simulink model "playback_data"  (R2015a)
settings: Solver=FixedStepDiscrete  SolverMode=SingleTasking  StartTime=76  StopTime=110  FixedStep=sample_time  RelTol=1e-3
undefined symbols (not defined in the file): A1_notch_f1, A2_notch_f1, A_kalman_swing_load, A_kalman_transverse, A_kalman_vertical, A_lpf_accelerometer, A_lpf_dtau, A_lpf_fourbar_angles, A_lpf_imu, A_lpf_lateral_angle, B1_lpf_accelerometer, B1_lpf_dtau, B1_lpf_fourbar_angles, B1_lpf_imu, B1_lpf_lateral_angle, B1_notch_f1, B2_lpf_accelerometer, B2_lpf_dtau, B2_lpf_fourbar_angles, B2_lpf_imu, B2_lpf_lateral_angle, B2_notch_f1, B_dx_versus_x0, B_kalman_swing_load, B_kalman_transverse, B_kalman_vertical, backwards_K_sag_of_t, backwards_P_sag_of_t, C_kalman_swing_load, C_kalman_transverse, C_kalman_vertical, com_leg_motor, com_torso, contact_threshold, control_start_time, d_ankle_to_foot, d_vertical_com, desired_com_forward_velocity, desired_com_lateral_velocity, desired_initial_leg_roll_left, desired_initial_leg_roll_right, desired_stance_beta2, desired_standing_torso_pitch, desired_standing_torso_roll, desired_standing_z, desired_torso_pitch, desired_torso_roll, Discrete, enable_bouncing, fcut_contact, fdesignblkfcn, forward_dx_of_dxstar, forward_x_of_dxstar, g, gcbh, HIP_MTR_MAX_CONT_TORQUE, HIP_MTR_MAX_TORQUE, i_leg_motor, i_robot, i_torso ... (+78)
libraries: simulink x65, dsparch4 x18, ctrlSharedLib x14, dspfdesign x4
(part 10 of 13)

== matlab function playback_data/Control/Actuator Control with Torque SEA commands/Detect Collision ==
  data: time input; spring_torque input; load_torque_derivative input; in_collision output; swing_collision_wait_time parameter
function in_collision = detect_collision(time, spring_torque, load_torque_derivative, swing_collision_wait_time)
    
    persistent collision_state time_of_collision;
    if isempty(collision_state)
        collision_state = logical(zeros(4,1));
        time_of_collision = zeros(4,1);
    end

    collision_detected = (abs(load_torque_derivative) > 2000 | abs(spring_torque) >= 50) & (time - time_of_collision > (1.5*swing_collision_wait_time));
    time_of_collision(collision_detected) = time;
    collision_state = collision_state | collision_detected;
    time_since_collision = time - time_of_collision;
    out_of_collision = (time_since_collision > swing_collision_wait_time) & (abs(spring_torque) < 50);
    collision_state(out_of_collision) = 0;
    %in_collision = collision_state;
    in_collision = [collision_state(1) | collision_state(2);
                    collision_state(1) | collision_state(2);
                    collision_state(3) | collision_state(4);
                    collision_state(3) | collision_state(4)];
    
end

== matlab function playback_data/Control/Actuator Control with Torque SEA commands/Load Torque Kalman Filter/MATLAB Function ==
  data: spring_torques input; R1 output; sample_time parameter; R2 output; R3 output; R4 output
function [R1, R2, R3, R4] = MeasurementCovariance(spring_torques, sample_time)
         
    high_torque_threshold = 80;
    low_torque_threshold = 50;
    high_deviation = 10;
    low_deviation = 0.1;
    
    deviation = (abs(spring_torques)-low_torque_threshold)*(low_deviation-high_deviation)/(high_torque_threshold-low_torque_threshold) + high_deviation;
    deviation(abs(spring_torques) <= low_torque_threshold) = high_deviation;
    deviation(abs(spring_torques) >= high_torque_threshold) = low_deviation;

    R1 = diag([(1e-6)^2, deviation(1)^2])/sample_time;
    R2 = diag([(1e-6)^2, deviation(2)^2])/sample_time;
    R3 = diag([(1e-6)^2, deviation(3)^2])/sample_time;
    R4 = diag([(1e-6)^2, deviation(4)^2])/sample_time;
end

== matlab function playback_data/Control/Actuator Control with Torque SEA commands/SEA Controller (Velocity)/Nonlinear Spring Force ==
  data: deflections input; tau_sea output
function tau_sea   = SeaSpringForce( deflections )
    tau_sea = SeaSpringForce( deflections );
end

== matlab function playback_data/Control/Behavior Control/Compute COM Translational Acceleration (IMU uses non-rotating measurement frame) ==
  data: com_acceleration_world output; torso_angular_accelerations input; imu_translational_accelerations_body input; torso_roll input; torso_pitch input; torso_yaw input; com_position_world input; com_velocity_world input; hip_roll_accelerations input; right_hip_roll input; left_hip_roll input; pelvis_to_imu parameter; com_torso parameter; com_leg_motor parameter; m_leg_motor parameter; m_leg parameter; m_torso parameter; torso_com_acceleration_world output; pelvis_acceleration_world output; right_hip_acceleration_world output; left_hip_acceleration_world output; com_acceleration_yawed output; g parameter
function [com_acceleration_world, torso_com_acceleration_world, pelvis_acceleration_world, right_hip_acceleration_world, left_hip_acceleration_world, com_acceleration_yawed] ...
          = compute_com_acceleration(torso_angular_accelerations, imu_translational_accelerations_body, torso_roll, torso_pitch, torso_yaw, ...
          com_position_world, com_velocity_world, ...
          hip_roll_accelerations, right_hip_roll, left_hip_roll, pelvis_to_imu, com_torso, com_leg_motor, m_leg_motor, m_leg, m_torso, g)

    % Body frame to Yawed frame rotations  
    R_body_to_yawed = R_pitch(torso_pitch(1))*R_roll(torso_roll(1));
    dR_body_to_yawed = dR_pitch(torso_pitch(1),torso_pitch(2))*R_roll(torso_roll(1)) + R_pitch(torso_pitch(1))*dR_roll(torso_roll(1),torso_roll(2));
    ddR_body_to_yawed = ddR_pitch(torso_pitch(1),torso_pitch(2),torso_angular_accelerations(2))*R_roll(torso_roll(1)) ...
                        + R_pitch(torso_pitch(1))*ddR_roll(torso_roll(1),torso_roll(2),torso_angular_accelerations(1)) ... 
                        + 2*dR_pitch(torso_pitch(1),torso_pitch(2))*dR_roll(torso_roll(1),torso_roll(2));
    % Yawed frame to World frame rotations  
    R_yawed_to_world = R_yaw(torso_yaw(1));
    dR_yawed_to_world = dR_yaw(torso_yaw(1),torso_yaw(2));
    ddR_yawed_to_world = ddR_yaw(torso_yaw(1),torso_yaw(2),torso_angular_accelerations(3));
    % Compute translational acceleration of torso COM
    R_position_body_to_world = R_yawed_to_world*R_body_to_yawed;
    R_velocity_body_to_world = dR_yawed_to_world*R_body_to_yawed + R_yawed_to_world*dR_body_to_yawed;
    R_acceleration_body_to_world = ddR_yawed_to_world*R_body_to_yawed + 2*dR_yawed_to_world*dR_body_to_yawed + R_yawed_to_world*ddR_body_to_yawed;
    imu_to_torso_com_acceleration_world = R_acceleration_body_to_world*(com_torso - pelvis_to_imu)';
    imu_acceleration_world = R_yawed_to_world*R_body_to_yawed*imu_translational_accelerations_body;
    torso_com_acceleration_world = imu_acceleration_world + imu_to_torso_com_acceleration_world;
    % Compute accelerations of hip COMs
    R_right_hip_to_body =     R_roll(-pi/2+right_hip_roll(1));
    dR_right_hip_to_body =   dR_roll(-pi/2+right_hip_roll(1), right_hip_roll(2));
    ddR_right_hip_to_body = ddR_roll(-pi/2+right_hip_roll(1), right_hip_roll(2), hip_roll_accelerations(1));
    R_left_hip_to_body =     R_roll(pi/2-left_hip_roll(1));
    dR_left_hip_to_body =   dR_roll(pi/2-left_hip_roll(1), -left_hip_roll(2));
    ddR_left_hip_to_body = ddR_roll(pi/2-left_hip_roll(1), -left_hip_roll(2), -hip_roll_accelerations(2));
    imu_to_pelvis_com_acceleration_world = R_acceleration_body_to_world*(-pelvis_to_imu)';  
    pelvis_acceleration_world = imu_acceleration_world + imu_to_pelvis_com_acceleration_world;
    left_hip_acceleration_world = pelvis_acceleration_world + (R_acceleration_body_to_world*R_left_hip_to_body + 2*R_velocity_body_to_world*dR_left_hip_to_body + R_position_body_to_world*ddR_left_hip_to_body)*com_leg_motor';
    right_hip_acceleration_world = pelvis_acceleration_world + (R_acceleration_body_to_world*R_right_hip_to_body + 2*R_velocity_body_to_world*dR_right_hip_to_body + R_position_body_to_world*ddR_right_hip_to_body)*(com_leg_motor.*[1,-1,1])';
    % Compute total system COM acceleration
    m_hip = m_leg+m_leg_motor;
    m_total = 2*m_hip + m_torso;
    com_acceleration_world = (m_torso*torso_com_acceleration_world + m_hip*(left_hip_acceleration_world + right_hip_acceleration_world))/m_total;
    com_acceleration_yawed = ddR_yawed_to_world'*com_position_world + 2*dR_yawed_to_world'*com_velocity_world + R_yawed_to_world'*com_acceleration_world;
    com_acceleration_yawed(3) = com_acceleration_yawed(3) - g;
end

function R_yp = R_pitch(theta) % map from pitched to yawed
  R_yp = [cos(theta), 0, sin(theta); ...
          0, 1, 0; ...
          -sin(theta), 0, cos(theta)];
end
function dR_yp = dR_pitch(theta,dtheta)
  dR_yp = dtheta*[-sin(theta), 0, cos(theta); ...
                  0, 0, 0; ... 
                  -cos(theta), 0, -sin(theta)];
end
function ddR_yp = ddR_pitch(theta,dtheta,ddtheta)
  ddR_yp = ddtheta*[-sin(theta), 0, cos(theta); ...
                    0, 0, 0; ... 
                    -cos(theta), 0, -sin(theta)] ...
           + dtheta^2*[-cos(theta), 0, -sin(theta); ...
                     0, 0, 0; ...
                     sin(theta), 0, -cos(theta)];
end
function R_pr = R_roll(phi) % map from rolled to pitched
  R_pr = [1, 0, 0; ...
          0, cos(phi), -sin(phi); ...
          0, sin(phi), cos(phi)]; 
end
function dR_pr = dR_roll(phi,dphi)
  dR_pr = dphi*[0, 0, 0; ...
                0, -sin(phi), -cos(phi); ...
                0, cos(phi), -sin(phi)];
end
function ddR_pr = ddR_roll(phi, dphi, ddphi)
  ddR_pr = ddphi*[0, 0, 0; ...
                  0, -sin(phi), -cos(phi); ...
                  0, cos(phi), -sin(phi)] ...
           + dphi^2*[0, 0, 0; ...
                   0, -cos(phi), sin(phi);...
                   0, -sin(phi), -cos(phi)];
end
function R_gy = R_yaw(psi) % map yawed frame to global
  R_gy = [cos(psi), -sin(psi), 0; sin(psi), cos(psi), 0; 0 0 1]; 
end
function dR_gy = dR_yaw(psi,dpsi)
  dR_gy = dpsi*[-sin(psi), -cos(psi), 0; cos(psi), -sin(psi), 0; 0 0 0];
end
function ddR_gy = ddR_yaw(psi,dpsi,ddpsi)
  ddR_gy = ddpsi*[-sin(psi), -cos(psi), 0; cos(psi), -sin(psi), 0; 0 0 0] ...
           + dpsi^2*[-cos(psi), sin(psi), 0; -sin(psi), -cos(psi), 0; 0 0 0];
end

== matlab function playback_data/Control/Behavior Control/Compute World Frame COM Coordinates from Yawed Frame ==
  data: com_position_world output; X_dX input; Y_dY input; Z_dZ input; torso_yaw input; com_velocity_world output
function [com_position_world, com_velocity_world] ...
          = compute_com_state_in_world_frame(X_dX, Y_dY, Z_dZ, torso_yaw)

    R_yawed_to_world = R_yaw(torso_yaw(1));
    dR_yawed_to_world = dR_yaw(torso_yaw(1),torso_yaw(2));
    
    com_position_yawed = [X_dX(1); Y_dY(1); Z_dZ(1)];
    com_velocity_yawed = [X_dX(2); Y_dY(2); Z_dZ(2)];
    
    com_position_world = R_yawed_to_world*com_position_yawed;
    com_velocity_world = dR_yawed_to_world*com_position_yawed + R_yawed_to_world*com_velocity_yawed;

end

function R_gy = R_yaw(psi) % map yawed frame to global
  R_gy = [cos(psi), -sin(psi), 0; sin(psi), cos(psi), 0; 0 0 1]; 
end
function dR_gy = dR_yaw(psi,dpsi)
  dR_gy = dpsi*[-sin(psi), -cos(psi), 0; cos(psi), -sin(psi), 0; 0 0 0];
end

== stateflow chart playback_data/Control/Behavior Control/Contact State Machine/State Machine ==
  state TouchDown
  state LockedContact
  state Unloading
  state Takeoff
  state Flight
  (junction 91) -> TouchDown
  TouchDown -> (junction 130) [order 2] : [vertical_grf < contact_threshold]
  (junction 93) -> (junction 91)
  (junction 130) -> (junction 128)
  TouchDown -> LockedContact [order 1] : [vertical_grf > loaded_threshold]
  (junction 115) -> LockedContact
  (junction 118) -> (junction 115)
  LockedContact -> Unloading : [z_velocity >= 0 && previous_z_velocity < 0]
  Unloading -> LockedContact [order 2] : [vertical_grf > loaded_threshold && z_velocity < 0]
  (junction 122) -> (junction 118)
  Unloading -> Takeoff [order 1] : [vertical_grf < contact_threshold]
  Takeoff -> Flight : after(t_flight,sec)
  (default) -> Flight
  Flight -> (junction 93) : [vertical_grf > contact_threshold]
  (junction 128) -> Flight
  data: z_velocity input; previous_z_velocity input; vertical_grf input; t_flight parameter; g parameter; contact_threshold parameter; loaded_threshold parameter; TouchDown output boolean; LockedContact output boolean; Unloading output boolean; Takeoff output boolean; Flight output boolean; vertical_acceleration input

== matlab function playback_data/Control/Behavior Control/Force Estimation/3D Forward Dynamics yawed ==
  data: right_or_left input; torso_roll input size=2; torso_pitch input double size=2; torso_yaw input double size=2; primary_sagittal_leg_angle input double size=2; primary_leg_length input double size=2; primary_leg_roll input double size=2; secondary_leg_roll input double size=2; primary_leg_torque input; primary_leg_force input; primary_lateral_torque input; secondary_lateral_torque input; R_GRF output double size=3; L_GRF output size=3; ddroll output double; g parameter; m_leg_motor parameter; m_torso parameter; i_torso parameter; i_leg_motor parameter; lateral_offset parameter; com_torso parameter; torso_centerline_roll_offset_angle parameter
%% Forward 3D ATRIAS dynamics
function [R_GRF, L_GRF, ddroll]  =  ForwardDynamics3D(right_or_left, ...
                                                      torso_roll, torso_pitch, torso_yaw, ...
                                                      primary_sagittal_leg_angle, primary_leg_length,...
                                                      primary_leg_roll, secondary_leg_roll, ...
                                                      primary_leg_torque, primary_leg_force, ...
                                                      primary_lateral_torque, secondary_lateral_torque, ...
                                                      g, m_leg_motor, m_torso, i_torso, i_leg_motor, lateral_offset, com_torso, torso_centerline_roll_offset_angle)

    d = norm(com_torso(2:3));
    It = mean(i_torso);
    Im = mean(i_leg_motor);
    
    phi    = torso_roll(1) + torso_centerline_roll_offset_angle;  % roll
    theta  = torso_pitch(1);                   % pitch
    alpha1 = primary_sagittal_leg_angle(1);    % primary sagittal leg angle
    beta1  = primary_leg_roll(1);              % primary leg roll
    beta2  = secondary_leg_roll(1);            % secondary leg roll
    if right_or_left
        beta1 = beta1 - torso_centerline_roll_offset_angle;
        beta2 = beta2 + torso_centerline_roll_offset_angle;
    else
        beta1 = beta1 + torso_centerline_roll_offset_angle;
        beta2 = beta2 - torso_centerline_roll_offset_angle;
    end 
    l1     = primary_leg_length(1);            % primary leg length
    
    dphi    = torso_roll(2);
    dtheta  = torso_pitch(2);
    dpsi    = torso_yaw(2);
    dalpha1 = primary_sagittal_leg_angle(2);
    dbeta1  = primary_leg_roll(2);
    dbeta2  = secondary_leg_roll(2);
    dl1     = primary_leg_length(2);
    
    
    tau_a1 = primary_leg_torque;
    tau_b1 = primary_lateral_torque;
    tau_b2 = secondary_lateral_torque;
    F_l1 = primary_leg_force;

    if right_or_left == 1
      A = A_fwd_yawed_right(lateral_offset,d,m_leg_motor,m_torso,It,Im,phi,theta,alpha1,beta1,beta2,l1);
      B = B_fwd_yawed_right(lateral_offset,d,g,m_leg_motor,m_torso,It,Im,phi,theta,alpha1,beta1,beta2,l1,dphi,dtheta,dpsi,dalpha1,dbeta1,dbeta2,dl1,tau_a1,tau_b1,tau_b2,F_l1);
    else
      A = A_fwd_yawed_left(lateral_offset,d,m_leg_motor,m_torso,It,Im,phi,theta,alpha1,beta1,beta2,l1);
      B = B_fwd_yawed_left(lateral_offset,d,g,m_leg_motor,m_torso,It,Im,phi,theta,alpha1,beta1,beta2,l1,dphi,dtheta,dpsi,dalpha1,dbeta1,dbeta2,dl1,tau_a1,tau_b1,tau_b2,F_l1);
    end
    
    x_fwd = A \ B;
    ddroll = x_fwd(4);
    GRF = zeros(3,1);
    GRF(1) = x_fwd(11);
    GRF(2) = x_fwd(12);
    GRF(3) = x_fwd(13); 
    
    if right_or_left == 1
        R_GRF = GRF;
        L_GRF = [0;0;0];
    else
        R_GRF = [0;0;0];
        L_GRF = GRF;
    end
end

== matlab function playback_data/Control1/Actuator Control with Torque SEA commands/Load Motion Disturbance Observer (Swing) Error-Proportional - 2nd order ==
  data: reset input; spring_torques input; d_hat_tp1 output size=[1 4]; positions input; velocities input; j_segments parameter; sample_time parameter
function d_hat_tp1  = disturbance_observer(reset, spring_torques, positions, velocities, j_segments, sample_time)

    order = 2;
    L = 2*2.^[1:order+1] .* factorial(order+1)./(factorial(order+1-(1:(order+1))).*factorial(1:order+1));
    N = 4;
    
    persistent z_t d_hat_t integral_term;
    if isempty(z_t)
        z_t = zeros(1,N);
        d_hat_t = zeros(1,N);
        integral_term = zeros(order,N);
    end
    
    for i=1:N
        if reset(i)
            z_t(i) = 0;
            d_hat_t(i) = 0;
            integral_term(:,i) = 0;
        end
    end
   
    % Define system
    A_d = [1, sample_time; 0, 1];
    Bu_d = [zeros(1,N); sample_time./j_segments];
    A_c = [0 1; 0 0];
    Bu_c = [zeros(1,N); 1./j_segments];
    Bd_c = [zeros(1,N); 1./j_segments];
    x = [positions'; velocities'];
    u = spring_torques;
 
    % Estimate disturbances
    z_tp1 = zeros(1,N);
    x_tp1 = zeros(2,N);
    d_hat_tp1 = zeros(1,N);
    for i=1:N
        z_tp1(i) = z_t(i) + sample_time*(pinv(Bd_c(:,i))*(A_c*x(:,i) + Bu_c(:,i)*u(i)) + d_hat_t(i));
        x_tp1(:,i) = A_d*x(:,i) + Bu_d(:,i)*u(i);
        integral_term(1,i) = integral_term(1,i) + sample_time*(pinv(Bd_c(:,i))*x_tp1(:,i) - z_tp1(i));
        for j=2:order
            integral_term(j,i) = integral_term(j,i) + sample_time*integral_term(j-1,i);
        end
        d_hat_tp1(i) = L*[(pinv(Bd_c(:,i))*x_tp1(:,i) - z_tp1(i)); integral_term(:,i)];
        d_hat_t(i) = d_hat_tp1(i);
        z_t(i) = z_tp1(i);
    end
    
end

== matlab function playback_data/Control/Behavior Control/Force Estimation/Leg Force Measurements/Nonlinear Spring Force ==
  data: deflections input; tau_sea output
function tau_sea   = SeaSpringForce( deflections )
    tau_sea = SeaSpringForce( deflections );
end

== matlab function playback_data/Control1/Actuator Control with Torque SEA commands/Load Torque Kalman Filter/MATLAB Function ==
  data: spring_torques input; R1 output; sample_time parameter; R2 output; R3 output; R4 output
function [R1, R2, R3, R4] = MeasurementCovariance(spring_torques, sample_time)
         
    high_torque_threshold = 80;
    low_torque_threshold = 50;
    high_deviation = 10;
    low_deviation = 0.1;
    
    deviation = (abs(spring_torques)-low_torque_threshold)*(low_deviation-high_deviation)/(high_torque_threshold-low_torque_threshold) + high_deviation;
    deviation(abs(spring_torques) <= low_torque_threshold) = high_deviation;
    deviation(abs(spring_torques) >= high_torque_threshold) = low_deviation;

    R1 = diag([(1e-6)^2, deviation(1)^2])/sample_time;
    R2 = diag([(1e-6)^2, deviation(2)^2])/sample_time;
    R3 = diag([(1e-6)^2, deviation(3)^2])/sample_time;
    R4 = diag([(1e-6)^2, deviation(4)^2])/sample_time;
end

== matlab function playback_data/Control1/Behavior Control/Compute World Frame COM Coordinates from Yawed Frame ==
  data: com_position_world output; X_dX input; Y_dY input; Z_dZ input; torso_yaw input; com_velocity_world output
function [com_position_world, com_velocity_world] ...
          = compute_com_state_in_world_frame(X_dX, Y_dY, Z_dZ, torso_yaw)

    R_yawed_to_world = R_yaw(torso_yaw(1));
    dR_yawed_to_world = dR_yaw(torso_yaw(1),torso_yaw(2));
    
    com_position_yawed = [X_dX(1); Y_dY(1); Z_dZ(1)];
    com_velocity_yawed = [X_dX(2); Y_dY(2); Z_dZ(2)];
    
    com_position_world = R_yawed_to_world*com_position_yawed;
    com_velocity_world = dR_yawed_to_world*com_position_yawed + R_yawed_to_world*com_velocity_yawed;

end

function R_gy = R_yaw(psi) % map yawed frame to global
  R_gy = [cos(psi), -sin(psi), 0; sin(psi), cos(psi), 0; 0 0 1]; 
end
function dR_gy = dR_yaw(psi,dpsi)
  dR_gy = dpsi*[-sin(psi), -cos(psi), 0; cos(psi), -sin(psi), 0; 0 0 0];
end

== stateflow chart playback_data/Control1/Behavior Control/Contact State Machine/State Machine ==
  state TouchDown
  state LockedContact
  state Unloading
  state Takeoff
  state Flight
  (junction 91) -> TouchDown
  TouchDown -> (junction 130) [order 2] : [vertical_grf < contact_threshold]
  (junction 93) -> (junction 91)
  (junction 130) -> (junction 128)
  TouchDown -> LockedContact [order 1] : [vertical_grf > loaded_threshold]
  (junction 115) -> LockedContact
  (junction 118) -> (junction 115)
  LockedContact -> Unloading : [z_velocity >= 0 && previous_z_velocity < 0]
  Unloading -> LockedContact [order 2] : [vertical_grf > loaded_threshold && z_velocity < 0]
  (junction 122) -> (junction 118)
  Unloading -> Takeoff [order 1] : [vertical_grf < contact_threshold]
  Takeoff -> Flight : after(t_flight,sec)
  (default) -> Flight
  Flight -> (junction 93) : [vertical_grf > contact_threshold]
  (junction 128) -> Flight
  data: z_velocity input; previous_z_velocity input; vertical_grf input; t_flight parameter; g parameter; contact_threshold parameter; loaded_threshold parameter; TouchDown output boolean; LockedContact output boolean; Unloading output boolean; Takeoff output boolean; Flight output boolean; vertical_acceleration input

== matlab function playback_data/Control1/Behavior Control/Force Estimation/3D Forward Dynamics yawed ==
  data: right_or_left input; torso_roll input size=2; torso_pitch input double size=2; torso_yaw input double size=2; primary_sagittal_leg_angle input double size=2; primary_leg_length input double size=2; primary_leg_roll input double size=2; secondary_leg_roll input double size=2; primary_leg_torque input; primary_leg_force input; primary_lateral_torque input; secondary_lateral_torque input; R_GRF output double size=3; L_GRF output size=3; ddroll output double; g parameter; m_leg_motor parameter; m_torso parameter; i_torso parameter; i_leg_motor parameter; lateral_offset parameter; com_torso parameter; torso_centerline_roll_offset_angle parameter
%% Forward 3D ATRIAS dynamics
function [R_GRF, L_GRF, ddroll]  =  ForwardDynamics3D(right_or_left, ...
                                                      torso_roll, torso_pitch, torso_yaw, ...
                                                      primary_sagittal_leg_angle, primary_leg_length,...
                                                      primary_leg_roll, secondary_leg_roll, ...
                                                      primary_leg_torque, primary_leg_force, ...
                                                      primary_lateral_torque, secondary_lateral_torque, ...
                                                      g, m_leg_motor, m_torso, i_torso, i_leg_motor, lateral_offset, com_torso, torso_centerline_roll_offset_angle)

    d = norm(com_torso(2:3));
    It = mean(i_torso);
    Im = mean(i_leg_motor);
    
    phi    = torso_roll(1) + torso_centerline_roll_offset_angle;  % roll
    theta  = torso_pitch(1);                   % pitch
    alpha1 = primary_sagittal_leg_angle(1);    % primary sagittal leg angle
    beta1  = primary_leg_roll(1);              % primary leg roll
    beta2  = secondary_leg_roll(1);            % secondary leg roll
    if right_or_left
        beta1 = beta1 - torso_centerline_roll_offset_angle;
        beta2 = beta2 + torso_centerline_roll_offset_angle;
    else
        beta1 = beta1 + torso_centerline_roll_offset_angle;
        beta2 = beta2 - torso_centerline_roll_offset_angle;
    end 
    l1     = primary_leg_length(1);            % primary leg length
    
    dphi    = torso_roll(2);
    dtheta  = torso_pitch(2);
    dpsi    = torso_yaw(2);
    dalpha1 = primary_sagittal_leg_angle(2);
    dbeta1  = primary_leg_roll(2);
    dbeta2  = secondary_leg_roll(2);
    dl1     = primary_leg_length(2);
    
    
    tau_a1 = primary_leg_torque;
    tau_b1 = primary_lateral_torque;
    tau_b2 = secondary_lateral_torque;
    F_l1 = primary_leg_force;

    if right_or_left == 1
      A = A_fwd_yawed_right(lateral_offset,d,m_leg_motor,m_torso,It,Im,phi,theta,alpha1,beta1,beta2,l1);
      B = B_fwd_yawed_right(lateral_offset,d,g,m_leg_motor,m_torso,It,Im,phi,theta,alpha1,beta1,beta2,l1,dphi,dtheta,dpsi,dalpha1,dbeta1,dbeta2,dl1,tau_a1,tau_b1,tau_b2,F_l1);
    else
      A = A_fwd_yawed_left(lateral_offset,d,m_leg_motor,m_torso,It,Im,phi,theta,alpha1,beta1,beta2,l1);
      B = B_fwd_yawed_left(lateral_offset,d,g,m_leg_motor,m_torso,It,Im,phi,theta,alpha1,beta1,beta2,l1,dphi,dtheta,dpsi,dalpha1,dbeta1,dbeta2,dl1,tau_a1,tau_b1,tau_b2,F_l1);
    end
    
    x_fwd = A \ B;
    ddroll = x_fwd(4);
    GRF = zeros(3,1);
    GRF(1) = x_fwd(11);
    GRF(2) = x_fwd(12);
    GRF(3) = x_fwd(13); 
    
    if right_or_left == 1
        R_GRF = GRF;
        L_GRF = [0;0;0];
    else
        R_GRF = [0;0;0];
        L_GRF = GRF;
    end
end

== matlab function playback_data/Control1/Behavior Control/Force Estimation/Leg Force Measurements/Nonlinear Spring Force ==
  data: deflections input; tau_sea output
function tau_sea   = SeaSpringForce( deflections )
    tau_sea = SeaSpringForce( deflections );
end

== matlab function playback_data/Control/Behavior Control/Knee Torques ==
  data: right_knees_to_foot input; right_front_knee_torques_from_fd output; left_knees_to_foot input; grf_from_seas input; grf_from_accelerometer input; right_back_knee_torques_from_fd output; right_front_knee_torques_from_accelerometer output; right_back_knee_torques_from_accelerometer output; left_front_knee_torques_from_fd output; left_back_knee_torques_from_fd output; left_front_knee_torques_from_accelerometer output; left_back_knee_torques_from_accelerometer output
function [right_front_knee_torques_from_fd, right_back_knee_torques_from_fd,...
          right_front_knee_torques_from_accelerometer, right_back_knee_torques_from_accelerometer,...
          left_front_knee_torques_from_fd, left_back_knee_torques_from_fd,...
          left_front_knee_torques_from_accelerometer, left_back_knee_torques_from_accelerometer] ...
          = compute_knee_torques(right_knees_to_foot, left_knees_to_foot, grf_from_seas, grf_from_accelerometer)

      right_front_knee_torques_from_fd = cross(right_knees_to_foot(1:3), grf_from_seas);
      right_back_knee_torques_from_fd = cross(right_knees_to_foot(4:6), grf_from_seas);
      right_front_knee_torques_from_accelerometer = cross(right_knees_to_foot(1:3), grf_from_accelerometer);
      right_back_knee_torques_from_accelerometer = cross(right_knees_to_foot(4:6), grf_from_accelerometer);
      
      left_front_knee_torques_from_fd = cross(left_knees_to_foot(1:3), grf_from_seas);
      left_back_knee_torques_from_fd = cross(left_knees_to_foot(4:6), grf_from_seas);
      left_front_knee_torques_from_accelerometer = cross(left_knees_to_foot(1:3), grf_from_accelerometer);
      left_back_knee_torques_from_accelerometer = cross(left_knees_to_foot(4:6), grf_from_accelerometer);
end

== matlab function playback_data/Control1/Behavior Control/Knee Torques ==
  data: right_knees_to_foot input; right_front_knee_torques_from_fd output; left_knees_to_foot input; grf_from_seas input; grf_from_accelerometer input; right_back_knee_torques_from_fd output; right_front_knee_torques_from_accelerometer output; right_back_knee_torques_from_accelerometer output; left_front_knee_torques_from_fd output; left_back_knee_torques_from_fd output; left_front_knee_torques_from_accelerometer output; left_back_knee_torques_from_accelerometer output
function [right_front_knee_torques_from_fd, right_back_knee_torques_from_fd,...
          right_front_knee_torques_from_accelerometer, right_back_knee_torques_from_accelerometer,...
          left_front_knee_torques_from_fd, left_back_knee_torques_from_fd,...
          left_front_knee_torques_from_accelerometer, left_back_knee_torques_from_accelerometer] ...
          = compute_knee_torques(right_knees_to_foot, left_knees_to_foot, grf_from_seas, grf_from_accelerometer)

      right_front_knee_torques_from_fd = cross(right_knees_to_foot(1:3), grf_from_seas);
      right_back_knee_torques_from_fd = cross(right_knees_to_foot(4:6), grf_from_seas);
      right_front_knee_torques_from_accelerometer = cross(right_knees_to_foot(1:3), grf_from_accelerometer);
      right_back_knee_torques_from_accelerometer = cross(right_knees_to_foot(4:6), grf_from_accelerometer);
      
      left_front_knee_torques_from_fd = cross(left_knees_to_foot(1:3), grf_from_seas);
      left_back_knee_torques_from_fd = cross(left_knees_to_foot(4:6), grf_from_seas);
      left_front_knee_torques_from_accelerometer = cross(left_knees_to_foot(1:3), grf_from_accelerometer);
      left_back_knee_torques_from_accelerometer = cross(left_knees_to_foot(4:6), grf_from_accelerometer);
end

== matlab function playback_data/Control1/Behavior Control/Primary Secondary Leg Swap/ToggleRightLeftLeg ==
  data: toggle input boolean; right_left output double; previous_right_left input double
function right_left = ToggleRightLeftLeg(toggle, previous_right_left)
    
    if toggle
        right_left = -previous_right_left + 1;
    else
        right_left = previous_right_left;
    end

end

== matlab function playback_data/Control1/Behavior Control/Primary and Lateral Behavior/Circular Buffer/Buffer ==
  data: data input; buffer output size=recorded_steps; trigger input; buffer_size input
function buffer  = buffer_data(data, trigger, buffer_size)

    persistent buffer_memory
    coder.varsize('buffer_memory',100);
    if isempty(buffer_memory)
        buffer_memory = [];
    end
    
    if trigger
        buffer_memory = [data; buffer_memory];
        if size(buffer_memory, 1) > buffer_size
            buffer_memory = buffer_memory(1:buffer_size,:);
        end
    end
    
    buffer = buffer_memory;

end

== matlab function playback_data/Control/Behavior Control/Primary Secondary Leg Swap/ToggleRightLeftLeg ==
  data: toggle input boolean; right_left output double; previous_right_left input double
function right_left = ToggleRightLeftLeg(toggle, previous_right_left)
    
    if toggle
        right_left = -previous_right_left + 1;
    else
        right_left = previous_right_left;
    end

end

== matlab function playback_data/Control1/Behavior Control/Primary and Lateral Behavior/Circular Buffer/Buffer1 ==
  data: data input; buffer output size=recorded_steps; trigger input; buffer_size input
function buffer  = buffer_data(data, trigger, buffer_size)

    persistent buffer_memory
    coder.varsize('buffer_memory',100);
    if isempty(buffer_memory)
        buffer_memory = [];
    end
    
    if trigger
        buffer_memory = [data; buffer_memory];
        if size(buffer_memory, 1) > buffer_size
            buffer_memory = buffer_memory(1:buffer_size,:);
        end
    end
    
    buffer = buffer_memory;

end

== matlab function playback_data/Control/Behavior Control/Primary and Lateral Behavior/Circular Buffer/Buffer ==
  data: data input; buffer output size=recorded_steps; trigger input; buffer_size input
function buffer  = buffer_data(data, trigger, buffer_size)

    persistent buffer_memory
    coder.varsize('buffer_memory',100);
    if isempty(buffer_memory)
        buffer_memory = [];
    end
    
    if trigger
        buffer_memory = [data; buffer_memory];
        if size(buffer_memory, 1) > buffer_size
            buffer_memory = buffer_memory(1:buffer_size,:);
        end
    end
    
    buffer = buffer_memory;

end

== matlab function playback_data/Control1/Behavior Control/Primary and Lateral Behavior/Circular Buffer/Buffer2 ==
  data: data input; buffer output size=recorded_steps; trigger input; buffer_size input
function buffer  = buffer_data(data, trigger, buffer_size)

    persistent buffer_memory
    coder.varsize('buffer_memory',100);
    if isempty(buffer_memory)
        buffer_memory = [];
    end
    
    if trigger
        buffer_memory = [data; buffer_memory];
        if size(buffer_memory, 1) > buffer_size
            buffer_memory = buffer_memory(1:buffer_size,:);
        end
    end
    
    buffer = buffer_memory;

end

== matlab function playback_data/Control1/Behavior Control/Primary and Lateral Behavior/Circular Buffer/Buffer3 ==
  data: data input; buffer output size=recorded_steps; trigger input; buffer_size input
function buffer  = buffer_data(data, trigger, buffer_size)

    persistent buffer_memory
    coder.varsize('buffer_memory',100);
    if isempty(buffer_memory)
        buffer_memory = [];
    end
    
    if trigger
        buffer_memory = [data; buffer_memory];
        if size(buffer_memory, 1) > buffer_size
            buffer_memory = buffer_memory(1:buffer_size,:);
        end
    end
    
    buffer = buffer_memory;

end

== matlab function playback_data/Control1/Behavior Control/Primary and Lateral Behavior/Circular Buffer/Buffer4 ==
  data: data input; buffer output size=recorded_steps; trigger input; buffer_size input
function buffer  = buffer_data(data, trigger, buffer_size)

    persistent buffer_memory
    coder.varsize('buffer_memory',100);
    if isempty(buffer_memory)
        buffer_memory = [];
    end
    
    if trigger
        buffer_memory = [data; buffer_memory];
        if size(buffer_memory, 1) > buffer_size
            buffer_memory = buffer_memory(1:buffer_size,:);
        end
    end
    
    buffer = buffer_memory;

end

== matlab function playback_data/Control1/Behavior Control/Primary and Lateral Behavior/Circular Buffer/Buffer5 ==
  data: data input; buffer output size=recorded_steps; trigger input; buffer_size input
function buffer  = buffer_data(data, trigger, buffer_size)

    persistent buffer_memory
    coder.varsize('buffer_memory',100);
    if isempty(buffer_memory)
        buffer_memory = [];
    end
    
    if trigger
        buffer_memory = [data; buffer_memory];
        if size(buffer_memory, 1) > buffer_size
            buffer_memory = buffer_memory(1:buffer_size,:);
        end
    end
    
    buffer = buffer_memory;

end

== matlab function playback_data/Control/Behavior Control/Primary and Lateral Behavior/Circular Buffer/Buffer1 ==
  data: data input; buffer output size=recorded_steps; trigger input; buffer_size input
function buffer  = buffer_data(data, trigger, buffer_size)

    persistent buffer_memory
    coder.varsize('buffer_memory',100);
    if isempty(buffer_memory)
        buffer_memory = [];
    end
    
    if trigger
        buffer_memory = [data; buffer_memory];
        if size(buffer_memory, 1) > buffer_size
            buffer_memory = buffer_memory(1:buffer_size,:);
        end
    end
    
    buffer = buffer_memory;

end

== matlab function playback_data/Control1/Behavior Control/Primary and Lateral Behavior/Circular Buffer/Buffer6 ==
  data: data input; buffer output size=recorded_steps; trigger input; buffer_size input
function buffer  = buffer_data(data, trigger, buffer_size)

    persistent buffer_memory
    coder.varsize('buffer_memory',100);
    if isempty(buffer_memory)
        buffer_memory = [];
    end
    
    if trigger
        buffer_memory = [data; buffer_memory];
        if size(buffer_memory, 1) > buffer_size
            buffer_memory = buffer_memory(1:buffer_size,:);
        end
    end
    
    buffer = buffer_memory;

end

== matlab function playback_data/Control/Behavior Control/Primary and Lateral Behavior/Circular Buffer/Buffer2 ==
  data: data input; buffer output size=recorded_steps; trigger input; buffer_size input
function buffer  = buffer_data(data, trigger, buffer_size)

    persistent buffer_memory
    coder.varsize('buffer_memory',100);
    if isempty(buffer_memory)
        buffer_memory = [];
    end
    
    if trigger
        buffer_memory = [data; buffer_memory];
        if size(buffer_memory, 1) > buffer_size
            buffer_memory = buffer_memory(1:buffer_size,:);
        end
    end
    
    buffer = buffer_memory;

end

== matlab function playback_data/Control/Behavior Control/Primary and Lateral Behavior/Circular Buffer/Buffer3 ==
  data: data input; buffer output size=recorded_steps; trigger input; buffer_size input
function buffer  = buffer_data(data, trigger, buffer_size)

    persistent buffer_memory
    coder.varsize('buffer_memory',100);
    if isempty(buffer_memory)
        buffer_memory = [];
    end
    
    if trigger
        buffer_memory = [data; buffer_memory];
        if size(buffer_memory, 1) > buffer_size
            buffer_memory = buffer_memory(1:buffer_size,:);
        end
    end
    
    buffer = buffer_memory;

end

== matlab function playback_data/Control/Behavior Control/Primary and Lateral Behavior/Circular Buffer/Buffer4 ==
  data: data input; buffer output size=recorded_steps; trigger input; buffer_size input
function buffer  = buffer_data(data, trigger, buffer_size)

    persistent buffer_memory
    coder.varsize('buffer_memory',100);
    if isempty(buffer_memory)
        buffer_memory = [];
    end
    
    if trigger
        buffer_memory = [data; buffer_memory];
        if size(buffer_memory, 1) > buffer_size
            buffer_memory = buffer_memory(1:buffer_size,:);
        end
    end
    
    buffer = buffer_memory;

end

== matlab function playback_data/Control/Behavior Control/Primary and Lateral Behavior/Circular Buffer/Buffer5 ==
  data: data input; buffer output size=recorded_steps; trigger input; buffer_size input
function buffer  = buffer_data(data, trigger, buffer_size)

    persistent buffer_memory
    coder.varsize('buffer_memory',100);
    if isempty(buffer_memory)
        buffer_memory = [];
    end
    
    if trigger
        buffer_memory = [data; buffer_memory];
        if size(buffer_memory, 1) > buffer_size
            buffer_memory = buffer_memory(1:buffer_size,:);
        end
    end
    
    buffer = buffer_memory;

end

== matlab function playback_data/Control/Behavior Control/Primary and Lateral Behavior/Circular Buffer/Buffer6 ==
  data: data input; buffer output size=recorded_steps; trigger input; buffer_size input
function buffer  = buffer_data(data, trigger, buffer_size)

    persistent buffer_memory
    coder.varsize('buffer_memory',100);
    if isempty(buffer_memory)
        buffer_memory = [];
    end
    
    if trigger
        buffer_memory = [data; buffer_memory];
        if size(buffer_memory, 1) > buffer_size
            buffer_memory = buffer_memory(1:buffer_size,:);
        end
    end
    
    buffer = buffer_memory;

end

== matlab function playback_data/Control/Behavior Control/Primary and Lateral Behavior/Circular Buffer/Buffer7 ==
  data: data input; buffer output size=recorded_steps; trigger input; buffer_size input
function buffer  = buffer_data(data, trigger, buffer_size)

    persistent buffer_memory
    coder.varsize('buffer_memory',100);
    if isempty(buffer_memory)
        buffer_memory = [];
    end
    
    if trigger
        buffer_memory = [data; buffer_memory];
        if size(buffer_memory, 1) > buffer_size
            buffer_memory = buffer_memory(1:buffer_size,:);
        end
    end
    
    buffer = buffer_memory;

end

== matlab function playback_data/Control/Behavior Control/Primary and Lateral Behavior/Closed Loop Compensation/CLOSED LOOP COMPENSATION X FOR VAIRABLE SPEED ==
  data: A_cl input; epsilon input; c input; delta_s_i input; dx_star input; B_cl input; delta_ux output
function delta_ux  = closed_loop_compensation_dxstar...
         (A_cl,epsilon, c, delta_s_i, dx_star, B_cl)
% assume form of delta_s_{i+1} = A_cl*delta_s_i + epsilon +c*dx_star + B_cl*delta_ux
% where delta measures deviation from deadbeat case. solve for
% delta_ux = (-A_cl*delta_s_i-epsilon - c*dxstar)/B_cl to achieve deadbeat
delta_ux = (-A_cl*delta_s_i - epsilon - c*dx_star)/B_cl;

== matlab function playback_data/Control1/Behavior Control/Primary and Lateral Behavior/Circular Buffer/Buffer7 ==
  data: data input; buffer output size=recorded_steps; trigger input; buffer_size input
function buffer  = buffer_data(data, trigger, buffer_size)

    persistent buffer_memory
    coder.varsize('buffer_memory',100);
    if isempty(buffer_memory)
        buffer_memory = [];
    end
    
    if trigger
        buffer_memory = [data; buffer_memory];
        if size(buffer_memory, 1) > buffer_size
            buffer_memory = buffer_memory(1:buffer_size,:);
        end
    end
    
    buffer = buffer_memory;

end

== matlab function playback_data/Control1/Behavior Control/Primary and Lateral Behavior/Closed Loop Compensation/CLOSED LOOP COMPENSATION X FOR VAIRABLE SPEED ==
  data: A_cl input; epsilon input; c input; delta_s_i input; dx_star input; B_cl input; delta_ux output
function delta_ux  = closed_loop_compensation_dxstar...
         (A_cl,epsilon, c, delta_s_i, dx_star, B_cl)
% assume form of delta_s_{i+1} = A_cl*delta_s_i + epsilon +c*dx_star + B_cl*delta_ux
% where delta measures deviation from deadbeat case. solve for
% delta_ux = (-A_cl*delta_s_i-epsilon - c*dxstar)/B_cl to achieve deadbeat
delta_ux = (-A_cl*delta_s_i - epsilon - c*dx_star)/B_cl;

== matlab function playback_data/Control1/Behavior Control/Primary and Lateral Behavior/Closed Loop Compensation/CLOSED LOOP COMPENSATION Y FOR VAIRABLE SPEED ==
  data: A_cl input; epsilon input; c input; delta_s_i input; dx_star input; B_cl input; delta_ux output
function delta_ux  = closed_loop_compensation_dxstar...
         (A_cl,epsilon, c, delta_s_i, dx_star, B_cl)
% assume form of delta_s_{i+1} = A_cl*delta_s_i + epsilon +c*dx_star + B_cl*delta_ux
% where delta measures deviation from deadbeat case. solve for
% delta_ux = (-A_cl*delta_s_i-epsilon - c*dxstar)/B_cl to achieve deadbeat
delta_ux = (-A_cl*delta_s_i - epsilon - c*dx_star)/B_cl;

== matlab function playback_data/Control1/Actuator Control with Torque SEA commands/SEA Controller (Velocity)/Nonlinear Spring Force ==
  data: deflections input; tau_sea output
function tau_sea   = SeaSpringForce( deflections )
    tau_sea = SeaSpringForce( deflections );
end

== matlab function playback_data/Control1/Behavior Control/Primary and Lateral Behavior/Closed Loop Compensation/ESTIMATE CLOSED LOOP ERROR X FOR VARIABLE SPEED ==
  data: dx_land_hist input; A_cl output; delta_ux_hist input; dx_lift_hist input; dx_star_hist input; B_dx_versus_x0 parameter; W_real input; epsilon_0 output; c output; A_cl_nb output; epsilon_0_nb output; c_nb output
function [A_cl, epsilon_0, c, ...
          A_cl_nb, epsilon_0_nb, c_nb] = error_fitting_dxstar...
         (dx_land_hist, delta_ux_hist, dx_lift_hist, dx_star_hist,...
          B_dx_versus_x0, W_real)
% data_length = min([length(dx_lift_hist), filter_length]);
data_length = length(dx_lift_hist);
assert(data_length < 100);
% add fake data
fake_dx_land_err_magnitude = 0.1; fake_dx_star_magnitude = 0.1;
[fgrid_dx_land_err, fgrid_dx_star, fgrid_dx_lift_err] = ...
    meshgrid(fake_dx_land_err_magnitude*[-1 1],fake_dx_star_magnitude*[-1 1],0);
fake_data_length = numel(fgrid_dx_land_err);
fake_dx_land_err = fgrid_dx_land_err(:);
fake_dx_star = fgrid_dx_star(:);
fake_dx_lift_err = fgrid_dx_lift_err(:);
fake_delta_ux = zeros(fake_data_length,1);
% assert(fake_data_length<100);
% assert(filter_length<100);
% fake_dx_land_err = linspace(-0.1, 0.1, fake_data_length)';
% fake_dx_lift_err = zeros(fake_data_length,1);
% fake_delta_ux = zeros(fake_data_length,1);
% fake_dx_star = linspace(-0.25, 0.25, fake_data_length)';
dx_land_err = [reshape(dx_land_hist(1:data_length)-dx_star_hist(1:data_length),...
                       data_length, 1); fake_dx_land_err];
dx_lift_err = [reshape(dx_lift_hist(1:data_length)-dx_star_hist(1:data_length),...
                       data_length, 1); fake_dx_lift_err];
dx_star = [reshape(dx_star_hist(1:data_length), data_length,1); fake_dx_star];
delta_ux = [reshape(delta_ux_hist(1:data_length), data_length, 1); fake_delta_ux];
% weighted least squares
W = diag([W_real*ones(1,data_length), ones(1,fake_data_length)]);
Y = dx_lift_err - B_dx_versus_x0*delta_ux;
X = [dx_land_err, dx_star, ones(data_length+fake_data_length,1)];
% linear regression for s_{i+1}-s0 = A_cl*(s_i-s0) + epsilon_0 + c(s0) + B*delta_u
% solve for Y = X*beta, beta column vector
beta_hat = (X'*W*X)\X'*W*Y;
W_nobias = diag([W_real*ones(1,data_length), 0.001*ones(1,fake_data_length)]);
beta_hat_nobias = (X'*W_nobias*X)\X'*W_nobias*Y;
A_cl = beta_hat(1);
c = beta_hat(2);
epsilon_0 = beta_hat(3);
A_cl_nb = beta_hat_nobias(1);
c_nb = beta_hat_nobias(2);
epsilon_0_nb = beta_hat_nobias(3);

== matlab function playback_data/Control/Behavior Control/Primary and Lateral Behavior/Closed Loop Compensation/CLOSED LOOP COMPENSATION Y FOR VAIRABLE SPEED ==
  data: A_cl input; epsilon input; c input; delta_s_i input; dx_star input; B_cl input; delta_ux output
function delta_ux  = closed_loop_compensation_dxstar...
         (A_cl,epsilon, c, delta_s_i, dx_star, B_cl)
% assume form of delta_s_{i+1} = A_cl*delta_s_i + epsilon +c*dx_star + B_cl*delta_ux
% where delta measures deviation from deadbeat case. solve for
% delta_ux = (-A_cl*delta_s_i-epsilon - c*dxstar)/B_cl to achieve deadbeat
delta_ux = (-A_cl*delta_s_i - epsilon - c*dx_star)/B_cl;

== matlab function playback_data/Control/Behavior Control/Primary and Lateral Behavior/Closed Loop Compensation/ESTIMATE CLOSED LOOP ERROR X FOR VARIABLE SPEED ==
  data: dx_land_hist input; A_cl output; delta_ux_hist input; dx_lift_hist input; dx_star_hist input; B_dx_versus_x0 parameter; W_real input; epsilon_0 output; c output; A_cl_nb output; epsilon_0_nb output; c_nb output
function [A_cl, epsilon_0, c, ...
          A_cl_nb, epsilon_0_nb, c_nb] = error_fitting_dxstar...
         (dx_land_hist, delta_ux_hist, dx_lift_hist, dx_star_hist,...
          B_dx_versus_x0, W_real)
% data_length = min([length(dx_lift_hist), filter_length]);
data_length = length(dx_lift_hist);
assert(data_length < 100);
% add fake data
fake_dx_land_err_magnitude = 0.1; fake_dx_star_magnitude = 0.1;
[fgrid_dx_land_err, fgrid_dx_star, fgrid_dx_lift_err] = ...
    meshgrid(fake_dx_land_err_magnitude*[-1 1],fake_dx_star_magnitude*[-1 1],0);
fake_data_length = numel(fgrid_dx_land_err);
fake_dx_land_err = fgrid_dx_land_err(:);
fake_dx_star = fgrid_dx_star(:);
fake_dx_lift_err = fgrid_dx_lift_err(:);
fake_delta_ux = zeros(fake_data_length,1);
% assert(fake_data_length<100);
% assert(filter_length<100);
% fake_dx_land_err = linspace(-0.1, 0.1, fake_data_length)';
% fake_dx_lift_err = zeros(fake_data_length,1);
% fake_delta_ux = zeros(fake_data_length,1);
% fake_dx_star = linspace(-0.25, 0.25, fake_data_length)';
dx_land_err = [reshape(dx_land_hist(1:data_length)-dx_star_hist(1:data_length),...
                       data_length, 1); fake_dx_land_err];
dx_lift_err = [reshape(dx_lift_hist(1:data_length)-dx_star_hist(1:data_length),...
                       data_length, 1); fake_dx_lift_err];
dx_star = [reshape(dx_star_hist(1:data_length), data_length,1); fake_dx_star];
delta_ux = [reshape(delta_ux_hist(1:data_length), data_length, 1); fake_delta_ux];
% weighted least squares
W = diag([W_real*ones(1,data_length), ones(1,fake_data_length)]);
Y = dx_lift_err - B_dx_versus_x0*delta_ux;
X = [dx_land_err, dx_star, ones(data_length+fake_data_length,1)];
% linear regression for s_{i+1}-s0 = A_cl*(s_i-s0) + epsilon_0 + c(s0) + B*delta_u
% solve for Y = X*beta, beta column vector
beta_hat = (X'*W*X)\X'*W*Y;
W_nobias = diag([W_real*ones(1,data_length), 0.001*ones(1,fake_data_length)]);
beta_hat_nobias = (X'*W_nobias*X)\X'*W_nobias*Y;
A_cl = beta_hat(1);
c = beta_hat(2);
epsilon_0 = beta_hat(3);
A_cl_nb = beta_hat_nobias(1);
c_nb = beta_hat_nobias(2);
epsilon_0_nb = beta_hat_nobias(3);

== matlab function playback_data/Control1/Behavior Control/Primary and Lateral Behavior/Closed Loop Compensation/ESTIMATE CLOSED LOOP ERROR Y FOR VARIABLE SPEED ==
  data: dx_land_hist input; A_cl output; delta_ux_hist input; dx_lift_hist input; dx_star_hist input; B_dx_versus_x0 parameter; W_real input; epsilon_0 output; c output; A_cl_nb output; epsilon_0_nb output; c_nb output
function [A_cl, epsilon_0, c, ...
          A_cl_nb, epsilon_0_nb, c_nb] = error_fitting_dxstar...
         (dx_land_hist, delta_ux_hist, dx_lift_hist, dx_star_hist,...
          B_dx_versus_x0, W_real)
% data_length = min([length(dx_lift_hist), filter_length]);
data_length = length(dx_lift_hist);
assert(data_length < 100);
% add fake data
fake_dx_land_err_magnitude = 0.1; fake_dx_star_magnitude = 0.1;
[fgrid_dx_land_err, fgrid_dx_star, fgrid_dx_lift_err] = ...
    meshgrid(fake_dx_land_err_magnitude*[-1 1],fake_dx_star_magnitude*[-1 1],0);
fake_data_length = numel(fgrid_dx_land_err);
fake_dx_land_err = fgrid_dx_land_err(:);
fake_dx_star = fgrid_dx_star(:);
fake_dx_lift_err = fgrid_dx_lift_err(:);
fake_delta_ux = zeros(fake_data_length,1);
% assert(fake_data_length<100);
% assert(filter_length<100);
% fake_dx_land_err = linspace(-0.1, 0.1, fake_data_length)';
% fake_dx_lift_err = zeros(fake_data_length,1);
% fake_delta_ux = zeros(fake_data_length,1);
% fake_dx_star = linspace(-0.25, 0.25, fake_data_length)';
dx_land_err = [reshape(dx_land_hist(1:data_length)-dx_star_hist(1:data_length),...
                       data_length, 1); fake_dx_land_err];
dx_lift_err = [reshape(dx_lift_hist(1:data_length)-dx_star_hist(1:data_length),...
                       data_length, 1); fake_dx_lift_err];
dx_star = [reshape(dx_star_hist(1:data_length), data_length,1); fake_dx_star];
delta_ux = [reshape(delta_ux_hist(1:data_length), data_length, 1); fake_delta_ux];
% weighted least squares
W = diag([W_real*ones(1,data_length), ones(1,fake_data_length)]);
Y = dx_lift_err - B_dx_versus_x0*delta_ux;
X = [dx_land_err, dx_star, ones(data_length+fake_data_length,1)];
% linear regression for s_{i+1}-s0 = A_cl*(s_i-s0) + epsilon_0 + c(s0) + B*delta_u
% solve for Y = X*beta, beta column vector
beta_hat = (X'*W*X)\X'*W*Y;
W_nobias = diag([W_real*ones(1,data_length), 0.001*ones(1,fake_data_length)]);
beta_hat_nobias = (X'*W_nobias*X)\X'*W_nobias*Y;
A_cl = beta_hat(1);
c = beta_hat(2);
epsilon_0 = beta_hat(3);
A_cl_nb = beta_hat_nobias(1);
c_nb = beta_hat_nobias(2);
epsilon_0_nb = beta_hat_nobias(3);
